simulink model "Step_3"  (R2024b)
settings: Solver=VariableStepAuto  StartTime=0.0  StopTime=100.0  RelTol=1e-3
libraries: dspsrcs4 x1
settings Model: Creator=Omar  LastModifiedBy=Omar

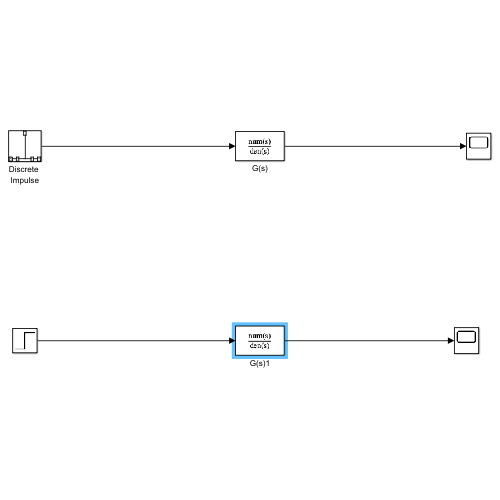
[thumbnail: Simulink's stored preview of the top-level diagram]
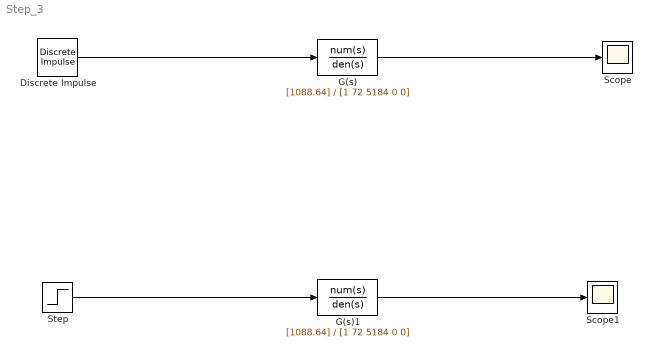
== system Step_3 ==
  Discrete Impulse : dspsrcs4/Discrete  Impulse  Delay=0  SampleTime=1  FrameSample=1  OutputFrames=off  dataType=double  isSigned=on  wordLen=16  udDataType=sfix(16)  fracBitsMode=Best precision  numFracBits=15  OutDataTypeStr=double  LastOutDataTypeStr=double
  G(s) : TransferFcn  Numerator=[1088.64]  Denominator=[1 72 5184 0 0]
  G(s)1 : TransferFcn  Numerator=[1088.64]  Denominator=[1 72 5184 0 0]
  Scope : Scope
  Scope1 : Scope
  Step : Step  SampleTime=0
  wires:
  Step/1 -> G(s)1/1
  G(s)1/1 -> Scope1/1
  G(s)/1 -> Scope/1
  Discrete Impulse/1 -> G(s)/1
